simulink library "ExternalChimes"  (R2022b)
settings: Solver=VariableStepAuto  StartTime=0.0  StopTime=10.0  RelTol=1e-3
values from neighbouring files (symbols this model uses):
  ext_chimes_rawSOS = zeros(ext_chimes_max_num_EQ_stages, 6)    [chimes_init.m]
undefined symbols (not defined in the file or in its folder): carModel, mode
libraries: TunableDelay x1, PooliirAccel x1, FeaturePath x1, TuneVar x1
settings Model: Creator=sc48041  LastModifiedBy=kl13806
settings SolverCC: AlgebraicLoopSolver=TrustRegion
settings DebuggingCC: UnconnectedInputMsg=warning  UnconnectedOutputMsg=warning  UnconnectedLineMsg=warning  SFMachineParentedDataDiag=warning
settings ModelReferenceCC: EnableRefExpFcnMdlSchedulingChecks=on
settings RTWCC: DLArmComputeVersion=19.05

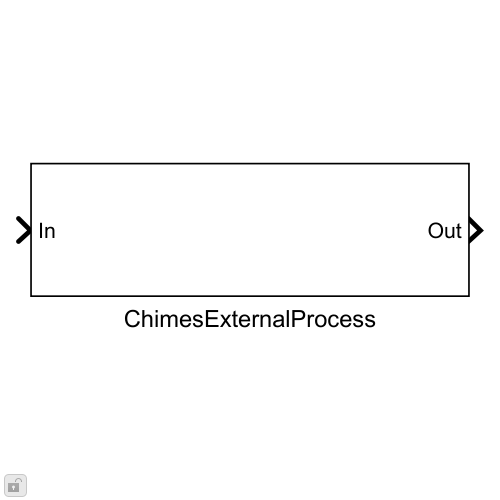
[thumbnail: Simulink's stored preview of the top-level diagram]
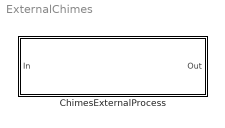
== system ExternalChimes ==
  ChimesExternalProcess : Subsystem

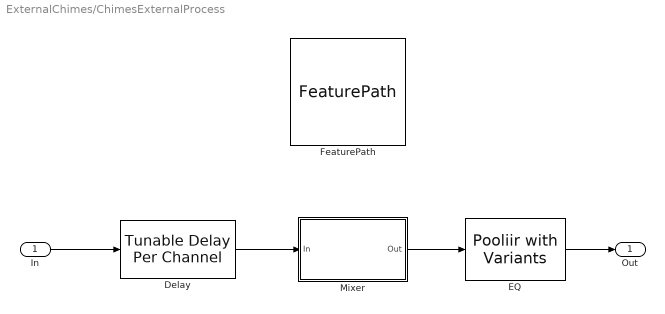
== system ExternalChimes/ChimesExternalProcess ==
  In : Inport
  Delay : TunableDelay/Tunable Delay Per Channel  FeatureName=Delay  maxDelayTime=ext_chimes_max_delay_in_samples  frameSize=frame_size  numChannels=NumExternalChimes  bufferAlias=[]  headerFilename=[]  MaskDelayType=In Samples  MaskValue=ext_chimes_init_delay
  EQ : PooliirAccel/Pooliir with Variants  variantSelect=Core  maxNumStages=ext_chimes_max_num_EQ_stages  numStages=ext_chime_numStages  sosCoefficients=single(ext_chimes_rawSOS)  frameSize=frame_size  numChannels=sys_defs.number_of_output_audio_channels  FeatureName=EQ
  FeaturePath : FeaturePath/FeaturePath  FeatureName=External  IsGroup=on  GroupNumber=5  DeclarePackages=on  PackageNames=mode,carModel  IsToolGroup=on  TriggerInit=[335 -156 450 -49]
  Mixer : Subsystem
  Out : Outport
  wires:
  EQ/1 -> Out/1
  Mixer/1(Out) -> EQ/1
  Delay/1 -> Mixer/1(In)
  In/1 -> Delay/1

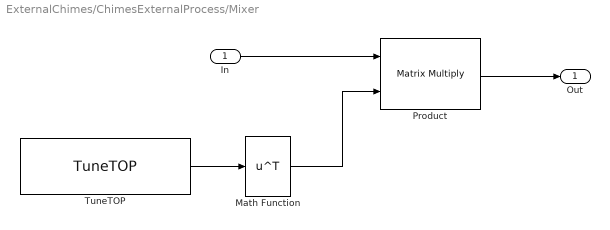
== system ExternalChimes/ChimesExternalProcess/Mixer ==
  In : Inport
  Math Function : Math  Operator=transpose  SignedPower=on
  Product : Product  Multiplication=Matrix(*)
  TuneTOP : TuneVar/TuneTOP  TriggerInit=[20 122 190 178]  TopName=MixerCoeff  TuneName=MixerCoeff  DataType=single  PackageName=mode  BankNumber=0  TunabilityNumber=1  MinValue=[]  MaxValue=[]  UseSameName=on  MaskValue=fMixerMatrixExtChimes
  Out : Outport
  wires:
  Math Function/1 -> Product/2
  TuneTOP/1 -> Math Function/1
  Product/1 -> Out/1
  In/1 -> Product/1
